simulink model "test_link_with_main_12"  (R2021b)
settings: Solver=ode15s  StartTime=0.0  StopTime=t_f  FixedStep=1  RelTol=1e-3
values from neighbouring files (symbols this model uses):
  waypoints = [0 0.5 0; 0.05 0.5 0 ... (first row only)    [manipulatorsim.m]    (also in manipulatorsim_UD.m)
  waypointVels = 0.002 *[ 0  0.05  0;0.05 0 0 ... (first row only)    [manipulatorsim.m]    (also in manipulatorsim_UD.m)
  waytime = 0:100:t_f    [manipulatorsim.m]    (also in manipulatorsim_UD.m)
libraries: robotmaniplib x1, robotcorelib x1
settings Model: Creator=Harish SG  LastModifiedBy=Harish SG
settings SolverCC: MaxOrder=2
settings ModelReferenceCC: ModelReferencePassRootInputsByReference=off

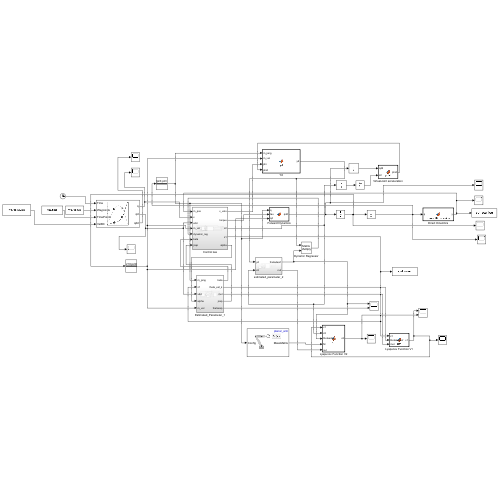
[thumbnail: Simulink's stored preview of the top-level diagram]
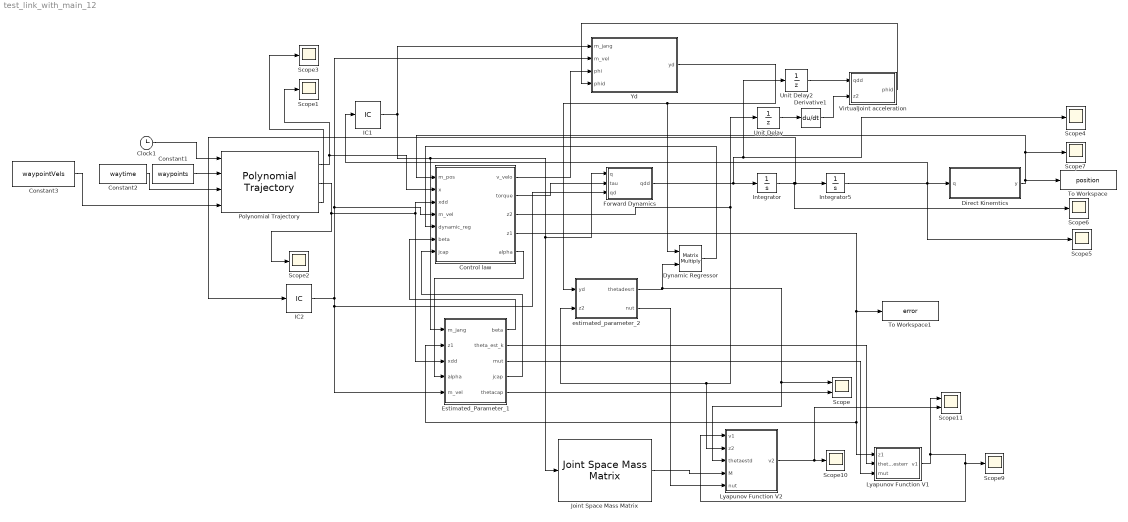
== system test_link_with_main_12 ==
  Clock1 : Clock
  Constant1 : Constant  Value=waypoints
  Constant2 : Constant  Value=waytime
  Constant3 : Constant  Value=waypointVels
  Control law : Subsystem
  Derivative1 : Derivative
  Direct Kinemtics : MATLAB Function  TreatAsAtomicUnit=on
  Dynamic Regressor : Product  Multiplication=Matrix(*)
  Estimated_Parameter_1 : Subsystem
  Forward Dynamics : MATLAB Function  TreatAsAtomicUnit=on
  IC1 : InitialCondition  Value=[pi/3;pi/3]
  IC2 : InitialCondition  Value=[pi/18;pi/20]
  Integrator : Integrator  InitialCondition=[pi/18;pi/20]  IgnoreLimit=on  ContinuousStateAttributes='acceleration'
  Integrator5 : Integrator  InitialCondition=[pi/3;pi/3]
  Joint Space Mass Matrix : robotmaniplib/Joint Space Mass Matrix  RigidBodyTree=planar_arm  SimulateUsing=Interpreted execution
  Lyapunov Function V1 : MATLAB Function  TreatAsAtomicUnit=on
  Lyapunov Function V2 : MATLAB Function  TreatAsAtomicUnit=on
  Polynomial Trajectory : robotcorelib/Polynomial Trajectory  WaypointSource=External  Waypoints=[ 0, 2, 1, 5, 0; -1, 3, 1, 4, 4 ]  TimePoints=[ 0, 1, 2, 3, 4 ]  TimeInterval=[ 1, 4 ]  Method=Cubic Polynomial  ParameterSource=External  VelocityBoundaryCondition=zeros( 2, 5 )  AccelerationBoundaryCondition=zeros( 2, 5 )  SimulateUsing=Interpreted execution
  Scope : Scope  NumInputPorts=2
  Scope{1..7,9..10} (9 alike) : Scope
  Scope11 : Scope  NumInputPorts=2
  To Workspace : ToWorkspace  VariableName=position  SaveFormat=Structure With Time  SampleTime=-1
  To Workspace1 : ToWorkspace  VariableName=error  SaveFormat=Structure With Time  SampleTime=-1
  Unit Delay : UnitDelay  SampleTime=-1  HasFrameUpgradeWarning=on
  Unit Delay2 : UnitDelay  SampleTime=-1  HasFrameUpgradeWarning=on
  VirtualJoint acceleration : MATLAB Function  TreatAsAtomicUnit=on
  Yd : MATLAB Function  TreatAsAtomicUnit=on
  estimated_parameter_2 : Subsystem
  wires:
  Clock1/1 -> Polynomial Trajectory/1
  Constant1/1 -> Polynomial Trajectory/2
  Constant2/1 -> Polynomial Trajectory/3
  Constant3/1 -> Polynomial Trajectory/4
  Polynomial Trajectory/1 -> Scope1/1, Control law/2(x)
  Polynomial Trajectory/3 -> Scope3/1
  Yd/1(yd) -> Dynamic Regressor/1, estimated_parameter_2/1(yd)
  Forward Dynamics/1(qdd) -> Integrator/1, Scope4/1, Unit Delay2/1
  IC2/1 -> Estimated_Parameter_1/5(m_vel), Forward Dynamics/3(qd), Yd/2(m_vel), Control law/4(m_vel)
  Integrator/1 -> Integrator5/1, IC2/1, Scope6/1
  IC1/1 -> Forward Dynamics/1(q), Joint Space Mass Matrix/1, Estimated_Parameter_1/1(m_jang), Yd/1(m_jang)
  Estimated_Parameter_1/4(jcap) -> Control law/7(jcap)
  estimated_parameter_2/1(thetadesrt) -> Scope/1, Lyapunov Function V2/3(thetaestd), Dynamic Regressor/2
  Polynomial Trajectory/2 -> Control law/3(xdd), Estimated_Parameter_1/3(xdd), Scope2/1
  Unit Delay/1 -> Derivative1/1
  Derivative1/1 -> VirtualJoint acceleration/2(z2)
  Unit Delay2/1 -> VirtualJoint acceleration/1(qdd)
  VirtualJoint acceleration/1(phid) -> Yd/4(phid)
  Estimated_Parameter_1/2(theta_est_k) -> Lyapunov Function V1/2(thetakesterr)
  Estimated_Parameter_1/3(mut) -> Lyapunov Function V1/3(mut)
  Joint Space Mass Matrix/1 -> Lyapunov Function V2/4(M)
  estimated_parameter_2/2(nut) -> Lyapunov Function V2/5(nut)
  Integrator5/1 -> Scope5/1, Direct Kinemtics/1(q), IC1/1
  Direct Kinemtics/1(y) -> Control law/1(m_pos), Scope7/1, To Workspace/1
  Lyapunov Function V1/1(v1) -> Lyapunov Function V2/1(v1), Scope9/1, Scope11/1
  Lyapunov Function V2/1(v2) -> Scope11/2, Scope10/1
  Estimated_Parameter_1/5(thetacap) -> Scope/2
  Control law/3(z2) -> Unit Delay/1, Lyapunov Function V2/2(z2), estimated_parameter_2/2(z2)
  Control law/4(z1) -> Estimated_Parameter_1/2(z1), Lyapunov Function V1/1(z1), To Workspace1/1
  Dynamic Regressor/1 -> Control law/5(dynamic_reg)
  Estimated_Parameter_1/1(beta) -> Control law/6(beta)
  Control law/1(v_velo) -> Yd/3(phi)
  Control law/2(torque) -> Forward Dynamics/2(tau)
  Control law/5(alpha) -> Estimated_Parameter_1/4(alpha)

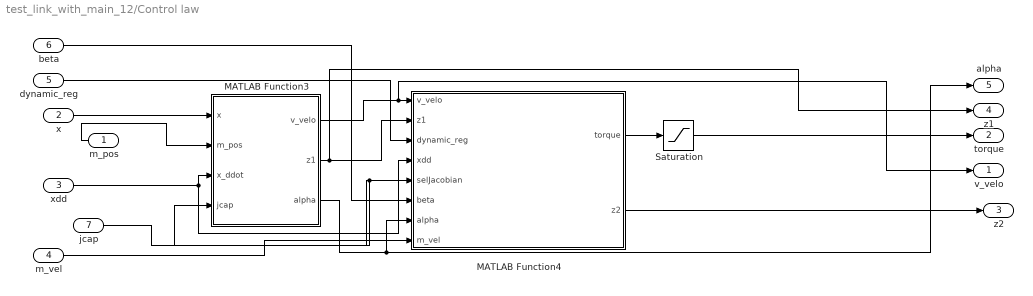
== system test_link_with_main_12/Control law ==
  m_pos : Inport
  x : Inport  Port=2
  xdd : Inport  Port=3
  m_vel : Inport  Port=4
  dynamic_reg : Inport  Port=5
  beta : Inport  Port=6
  jcap : Inport  Port=7
  MATLAB Function3 : MATLAB Function  TreatAsAtomicUnit=on
  MATLAB Function4 : MATLAB Function  TreatAsAtomicUnit=on
  Saturation : Saturate  UpperLimit=[5,5]  LowerLimit=[0.0001,0.0001]
  v_velo : Outport
  torque : Outport  Port=2
  z2 : Outport  Port=3
  z1 : Outport  Port=4
  alpha : Outport  Port=5
  wires:
  beta/1 -> MATLAB Function4/6(beta)
  MATLAB Function4/1(torque) -> Saturation/1
  Saturation/1 -> torque/1
  MATLAB Function3/1(v_velo) -> v_velo/1, MATLAB Function4/1(v_velo)
  MATLAB Function3/3(alpha) -> alpha/1, MATLAB Function4/7(alpha)
  xdd/1 -> MATLAB Function4/4(xdd), MATLAB Function3/3(x_ddot)
  MATLAB Function4/2(z2) -> z2/1
  x/1 -> MATLAB Function3/1(x)
  jcap/1 -> MATLAB Function4/5(selJacobian), MATLAB Function3/4(jcap)
  dynamic_reg/1 -> MATLAB Function4/3(dynamic_reg)
  MATLAB Function3/2(z1) -> z1/1, MATLAB Function4/2(z1)
  m_pos/1 -> MATLAB Function3/2(m_pos)
  m_vel/1 -> MATLAB Function4/8(m_vel)

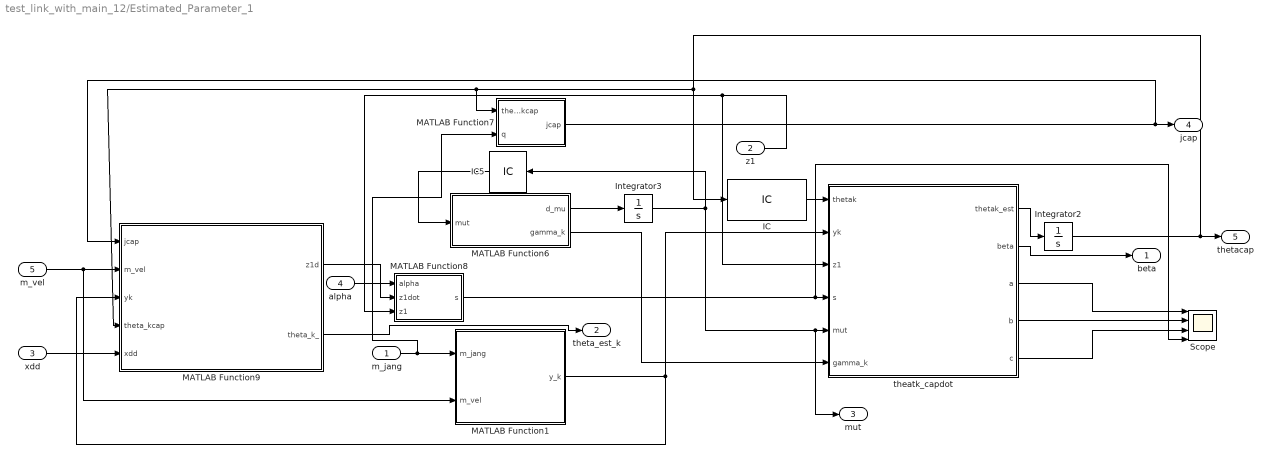
== system test_link_with_main_12/Estimated_Parameter_1 ==
  m_jang : Inport
  z1 : Inport  Port=2
  xdd : Inport  Port=3
  alpha : Inport  Port=4
  m_vel : Inport  Port=5
  " theatk_capdot" : MATLAB Function  TreatAsAtomicUnit=on
  IC : InitialCondition  Value=[0.35;0.35]
  IC5 : InitialCondition  Value=[0.01;0.01]
  Integrator2 : Integrator  InitialCondition=[0.35;0.35]
  Integrator3 : Integrator  InitialCondition=[0.01;0.01]
  MATLAB Function1 : MATLAB Function  TreatAsAtomicUnit=on
  MATLAB Function6 : MATLAB Function  TreatAsAtomicUnit=on
  MATLAB Function7 : MATLAB Function  TreatAsAtomicUnit=on
  MATLAB Function8 : MATLAB Function  TreatAsAtomicUnit=on
  MATLAB Function9 : MATLAB Function  TreatAsAtomicUnit=on
  Scope : Scope  NumInputPorts=4
  beta : Outport
  theta_est_k : Outport  Port=2
  mut : Outport  Port=3
  jcap : Outport  Port=4
  thetacap : Outport  Port=5
  wires:
  MATLAB Function6/1(d_mu) -> Integrator3/1
  m_jang/1 -> MATLAB Function7/2(q), MATLAB Function1/1(m_jang)
  MATLAB Function1/1(y_k) -> MATLAB Function9/3(yk), " theatk_capdot"/2(yk)
  MATLAB Function9/1(z1d) -> MATLAB Function8/2(z1dot)
  m_vel/1 -> MATLAB Function1/2(m_vel), MATLAB Function9/2(m_vel)
  z1/1 -> MATLAB Function8/3(z1), " theatk_capdot"/3(z1)
  MATLAB Function8/1(s) -> Scope/4, " theatk_capdot"/4(s)
  MATLAB Function6/2(gamma_k) -> " theatk_capdot"/6(gamma_k)
  MATLAB Function7/1(jcap) -> jcap/1, MATLAB Function9/1(jcap)
  " theatk_capdot"/1(thetak_est) -> Integrator2/1
  " theatk_capdot"/2(beta) -> beta/1
  Integrator3/1 -> mut/1, " theatk_capdot"/5(mut), IC5/1
  xdd/1 -> MATLAB Function9/5(xdd)
  alpha/1 -> MATLAB Function8/1(alpha)
  MATLAB Function9/2(theta_k_) -> theta_est_k/1
  IC/1 -> " theatk_capdot"/1(thetak)
  Integrator2/1 -> thetacap/1, MATLAB Function9/4(theta_kcap), MATLAB Function7/1(thetakcap), IC/1
  IC5/1 -> MATLAB Function6/1(mut)
  " theatk_capdot"/3(a) -> Scope/1
  " theatk_capdot"/4(b) -> Scope/2
  " theatk_capdot"/5(c) -> Scope/3

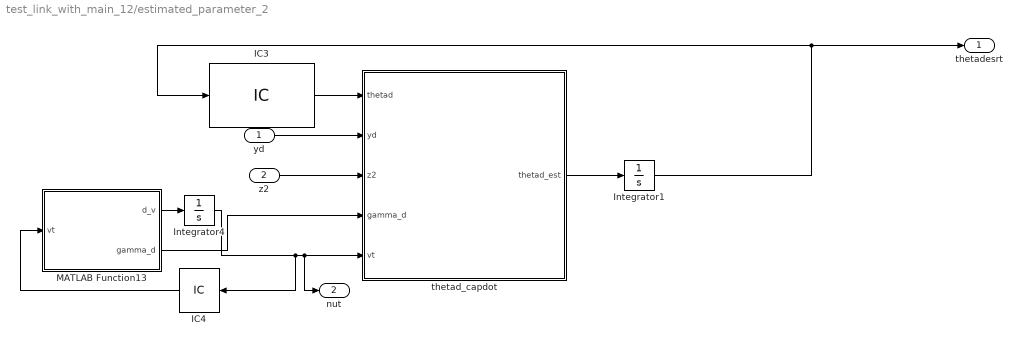
== system test_link_with_main_12/estimated_parameter_2 ==
  yd : Inport
  z2 : Inport  Port=2
  IC3 : InitialCondition  Value=[1.2;1.2;1.2;1.2;1.2;1.2;1.2;1.2]
  IC4 : InitialCondition  Value=0.001*[1;1;1;1;1;1;1;1]
  Integrator1 : Integrator  InitialCondition=[1.2;1.2;1.2;1.2;1.2;1.2;1.2;1.2]
  Integrator4 : Integrator  InitialCondition=0.001*[1;1;1;1;1;1;1;1]
  MATLAB Function13 : MATLAB Function  TreatAsAtomicUnit=on
  thetad_capdot : MATLAB Function  TreatAsAtomicUnit=on
  thetadesrt : Outport
  nut : Outport  Port=2
  wires:
  MATLAB Function13/2(gamma_d) -> thetad_capdot/4(gamma_d)
  thetad_capdot/1(thetad_est) -> Integrator1/1
  MATLAB Function13/1(d_v) -> Integrator4/1
  yd/1 -> thetad_capdot/2(yd)
  Integrator1/1 -> IC3/1, thetadesrt/1
  Integrator4/1 -> IC4/1, nut/1, thetad_capdot/5(vt)
  z2/1 -> thetad_capdot/3(z2)
  IC3/1 -> thetad_capdot/1(thetad)
  IC4/1 -> MATLAB Function13/1(vt)

== matlab function test_link_with_main_12/Estimated_Parameter_1/MATLAB Function8 ==
  data: alpha input; s output; z1dot input; z1 input
function s = s(alpha,z1dot,z1)

s = z1dot+(alpha*z1);

== matlab function test_link_with_main_12/Estimated_Parameter_1/MATLAB Function9 ==
  data: jcap input; z1d output; m_vel input; yk input; theta_kcap input; xdd input; theta_k_ output
function [z1d,theta_k_] = z1d(jcap, m_vel, yk, theta_kcap, xdd)
l2 = 0.31;
l1 = 0.3;
theta_k = [l1;l2];
theta_k_ = theta_k - theta_kcap;
z1d = (jcap*m_vel)+(yk*theta_k_) - xdd(1:2,:);

== matlab function test_link_with_main_12/Yd ==
  data: m_jang input; yd output; m_vel input; phi input; phid input
function yd = yd(m_jang,m_vel,phi,phid)
 q1 = m_jang(1);
 q2 = m_jang(2);
 qd1 = m_vel(1);
 qd2 = m_vel(2);
 pi1 = phi(1);
 pi2 = phi(2);
pid1= phid(1);
pid2= phid(2);
l1 = 0.3;
l2 = 0.31;g = -9.8;
y11 = l1^2*pid1+l1*g*cos(q1);
y12 = 2*l1*pid1+g*cos(q1);
y13 = pid1;
y14 =0;
y15 =(l1^2+2*l1*l2*cos(q2)+l2^2)*pid1+((l1*l2*cos(q2)+l2^2)*pid2)- (2*l1*l2*sin(q2)*qd1*pi2)-(l1*l2*sin(q2)*pi2*qd2)+(l1*g*cos(q1))+(l2*g*cos(q1+q2));
y16 = (2*l1*cos(q2)+2*l2)*pid1+(l1*cos(q1)+2*l2)*pid2 - 2*l1*sin(q2)*qd1*qd2 -l1*sin(q2)*qd2*pi2+g*cos(q1+q2);
y17 = pid1+pid2;
y18 = 0;
y21 = 0;
y22 = 0;
y23 = 0;
y24 = 0;
y25 = ((l1*l2*cos(q2)+l2^2)*pid1)+(l2^2*pid2)+(l1*l2*sin(q2)*pi1*qd1)+(l2*g*cos(q1+q2));
y26 = (l1*cos(q2)+2*l2)*pid1+2*l2*pid2+l1*sin(q2)*qd1*pi1+g*cos(q1+q2);
y27 = pid1+pid2;
y28 = 0;
yd = [y11,y12,y13,y14,y15,y16,y17,y18;
    y21,y22,y23,y24,y25,y26,y27,y28];

== matlab function test_link_with_main_12/estimated_parameter_2/thetad_capdot ==
  data: thetad input; thetad_est output; yd input; z2 input; gamma_d input; vt input
function thetad_est = thetad_capdot(thetad,yd,z2,gamma_d,vt)

ydtrans = yd';

thetad_est =-gamma_d*(ydtrans*z2) - diag(vt) * thetad;

== matlab function test_link_with_main_12/Lyapunov Function V1 ==
  data: z1 input; v1 output; thetakesterr input; mut input
function v1  = clfh(z1,thetakesterr,mut)
z = (z1'*z1)/2;
thetak = [0.3;0.31];
igk = inv([3 0; 0 3]);
li = ((thetakesterr')*igk*thetakesterr);
ci = (thetak'*diag(mut)*thetak);
v1 = z+li+ci;

== matlab function test_link_with_main_12/estimated_parameter_2/MATLAB Function13 ==
  data: vt input; d_v output; gamma_d output
function [d_v,gamma_d] = d_v(vt)
a =400;
gamma_d = a*eye(8);
ingammad = inv(gamma_d);
d_v = -(ingammad*vt);

== matlab function test_link_with_main_12/Lyapunov Function V2 ==
  data: v1 input; v2 output; z2 input; thetaestd input; M input; nut input
function v2  = fcn(v1,z2,thetaestd,M,nut)
m1 = 1; m2 =1;
l1 = 0.3; l2 = 0.31;a1 = 0.15; a2 = 0.15;


a= (z2')*M*z2;
gammad = 400*eye(8);
igd = inv(gammad);
b = (thetaestd')*igd*thetaestd;
t1 = m1;
t2 = m2*(a1-l1);
t3 = m1*(a1-l1)^2;
t5 = m2;
t6 = m2*(a2-l2);
t7 = m2*(a2-l2)^2;
t8 =0;
thetad = [t1;t2;t3;0;t5;t6;t7;t8];
c = (thetad')*diag(nut)*thetad;
v2 = v1+a+b+c;

== matlab function test_link_with_main_12/Forward Dynamics ==
  data: q input; qdd output; tau input; qd input
function qdd = fd(q,tau,qd)
theta1 = q(1);
theta2 = q(2);
qd1 = qd(1);
qd2 = qd(2);
m1 = 1; m2 = 1; l1 = 0.3; l2 = 0.31; a1 = .15;
a2 = .15; g = -9.81;I1 = 0;
 I2 =0;
% mass matrix from joint space equation of motion
M = [m1*(a1^2)+I1+I2+m2*((a2^2)+(l1^2)+(2*l1*a2*cos(theta2))) I2+m2*((a2^2)+(l1*a2*cos(theta2)));I2+m2*((a2^2)+(l1*a2*cos(theta2))) m2*(a2^2)+I2];
vq = [(-2*m2*a2*l1*sin(theta2)*qd1*qd2)-m2*a2*l1*sin(theta2)*(qd2)^2;m2*a2*l1*sin(theta2)*qd2];
Gq = [g*(m2*(a2*cos(theta1 + theta2) + l1*cos(theta1)) + l1*m1*cos(theta1)); a2*g*m2*cos(theta1 + theta2)];
Minv = inv(M);
qdd = -Minv*(vq) - Minv*(Gq)+tau;

== matlab function test_link_with_main_12/Estimated_Parameter_1/MATLAB Function1 ==
  data: m_jang input; y_k output; m_vel input
function y_k = yk(m_jang,m_vel)
     q1 = m_jang(1);
     q2 = m_jang(2);
     qd1 = m_vel(1);
     qd2 = m_vel(2);
     s12 = (sin(q1)*cos(q2))+(cos(q1)*sin(q2));
c12 = (cos(q1)*cos(q2))-(sin(q1)*sin(q2));
      y_k = [-sin(q1)*qd1, -s12*(qd1+qd2);
          cos(q1)*qd1, c12*(qd1+qd2)];

== matlab function test_link_with_main_12/VirtualJoint acceleration ==
  data: qdd input; phid output; z2 input
function phid = phid(qdd,z2)
phid = qdd-z2;

== matlab function test_link_with_main_12/Estimated_Parameter_1/ theatk_capdot ==
  data: thetak input; thetak_est output; yk input; z1 input; s input; mut input; beta output; gamma_k input; a output; b output; c output
function [thetak_est,beta,a,b,c] = thetak_capdot(thetak,yk,z1,s,mut,gamma_k)
beta = 2;
%A = 2*eye(2);
%x = [0.3;0.31];
%thetak_est = -A*x;
yktrans = yk';

 a  =  gamma_k*(yktrans*z1);
 b =  gamma_k*(2*beta*yktrans*s);
 c = diag(mut)* thetak;
 thetak_est = a+b-c;

== matlab function test_link_with_main_12/Control law/MATLAB Function3 ==
  data: x input; v_velo output; m_pos input; x_ddot input; z1 output; jcap input; alpha output
function [v_velo,z1,alpha] = virtControl(x,m_pos,x_ddot,jcap)
alpha =0.01;
ijcap = inv(jcap);    
z1 = m_pos - x(1:2,:);
eie = - (alpha*z1)+x_ddot(1:2,:) ;
v_velo = ijcap*eie;%inv(jcap)*(- (alpha*z1)+x_ddot(1:2,:)) since the matlab threw a warning

== matlab function test_link_with_main_12/Control law/MATLAB Function4 ==
  data: v_velo input; z1 input; dynamic_reg input; xdd input; torque output; selJacobian input; beta input; alpha input; z2 output; m_vel input
function [torque, z2] = sysControl(v_velo, z1, dynamic_reg, xdd, selJacobian, beta, alpha, m_vel)
eta =100;
scap = selJacobian*m_vel-xdd(1:2,:)+alpha*z1; 
z2 = m_vel - v_velo;
torque =  -((selJacobian')*z1) -(beta*(selJacobian')*scap) - (eta*z2)+dynamic_reg ;

== matlab function test_link_with_main_12/Direct Kinemtics ==
  data: q input; y output
function y = forwardKinematics(q)
 q1 = q(1);
 q2 = q(2);
 l1 = 0.3; l2 =0.31;
s12 = (sin(q1)*cos(q2))+(cos(q1)*sin(q2));
 c11= (cos(q1)*cos(q2))-(sin(q1)*sin(q2));
 y = [ l1*cos(q1) + l2*c11 ;...
          l1*sin(q1) + l2*s12 ];

== matlab function test_link_with_main_12/Estimated_Parameter_1/MATLAB Function6 ==
  data: mut input; d_mu output; gamma_k output
function [d_mu,gamma_k] = d_mu(mut)

gamma_k = 3*eye(2);
ingammak = inv(gamma_k);
d_mu = -(ingammak*mut);

== matlab function test_link_with_main_12/Estimated_Parameter_1/MATLAB Function7 ==
  data: thetakcap input; jcap output; q input
function jcap = Jcap(thetakcap,q)
a1 = thetakcap(1);
a2 = thetakcap(2);
q1 =q(1);
q2 =q(2);
jcap = [-(a1*sin(q1)+a2*sin(q1+q2)), -(a2*sin(q1+q2)); 
    (a1*cos(q1)+a2*cos(q1+q2)), (a2*cos(q1+q2))];
